simulink model "ZuflussAbfluss1"  (Simulink 7.1)
settings: Solver=ode45  StartTime=0.0  StopTime=10.0  RelTol=1e-3
settings Model: Creator=Meisel  LastModifiedBy=Meisel

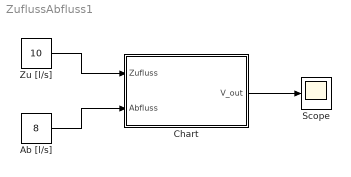
== system ZuflussAbfluss1 ==
  Ab [l/s] : Constant  Value=8  OutDataType=sfix(16)  OutScaling=2^0
  Chart : Stateflow chart
  Scope : Scope
  Zu [l/s] : Constant  Value=10  OutDataType=sfix(16)  OutScaling=2^0
  wires:
  Chart/1(V_out) -> Scope/1
  Zu [l/s]/1 -> Chart/1(Zufluss)
  Ab [l/s]/1 -> Chart/2(Abfluss)

== stateflow chart Chart ==
  settings: updateMethod=CONTINUOUS
  state Fill
    during:
    // derivatives (Ableitungen)
    V_dot=Zufluss-Abfluss;
    // output
    V_out = V;
  (default) -> Fill : {V=0;}
  data: Zufluss input double; Abfluss input double; V_out output double; V local double
  data V settings: updateMethod=SF_CONTINUOUS_TIME_DATA
